simulink model "ADCS"  (R2018b)
settings: Solver=VariableStepAuto  StartTime=0.0  StopTime=10  RelTol=1e-3
undefined symbols (not defined in the file): f, Jw, Kb, km, Kt, La, N, Ra, tau
libraries: vrlib x1
settings Model: Creator=mario  LastModifiedBy=mario

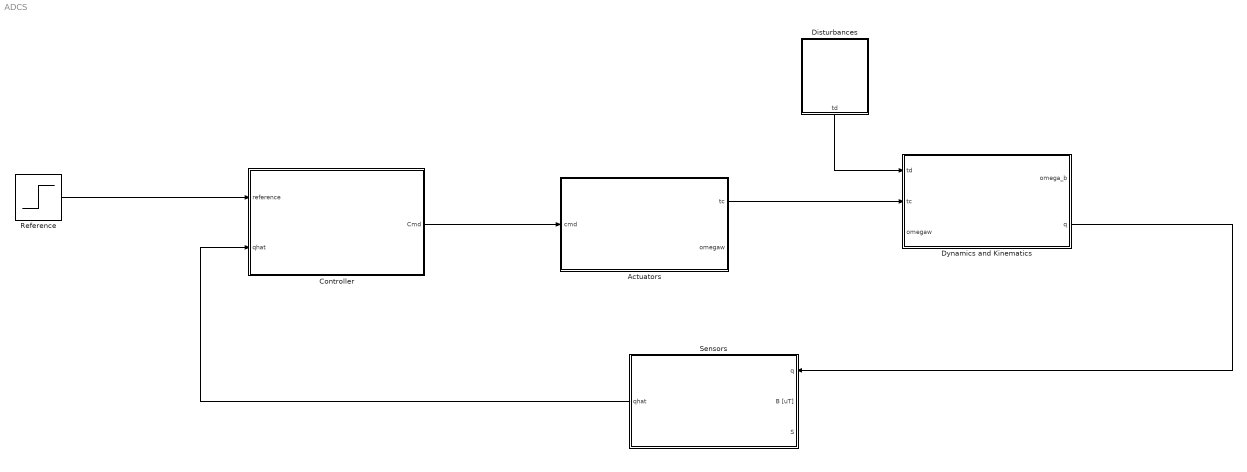
== system ADCS ==
  Actuators : Subsystem
  Controller : Subsystem
  Disturbances : Subsystem
  "Dynamics and Kinematics " : Subsystem
  Reference : Step  SampleTime=0
  Sensors : Subsystem
  wires:
  "Dynamics and Kinematics "/2(q) -> Sensors/1(q)
  Sensors/1(qhat) -> Controller/2(qhat)
  Controller/1(Cmd) -> Actuators/1(cmd)
  Disturbances/1(td) -> "Dynamics and Kinematics "/1(td)
  Actuators/1(tc) -> "Dynamics and Kinematics "/2(tc)
  Reference/1 -> Controller/1("reference ")

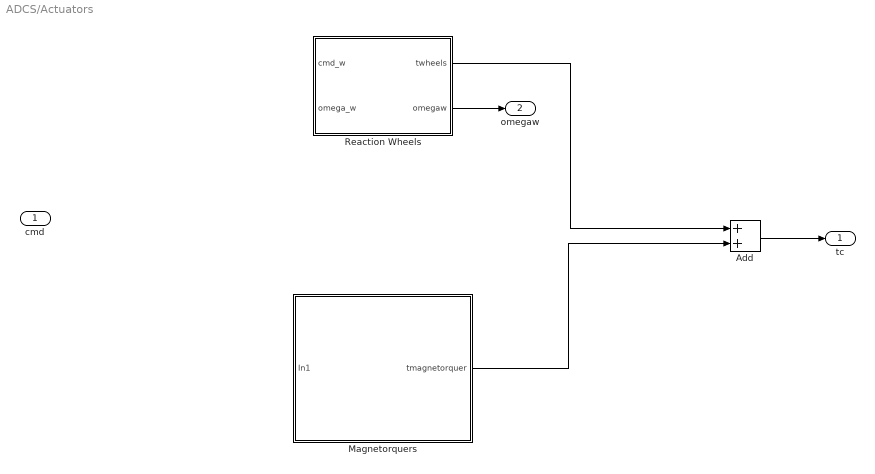
== system ADCS/Actuators ==
  cmd : Inport
  Add : Sum
  Magnetorquers : Subsystem
  Reaction Wheels : Subsystem
  tc : Outport
  omegaw : Outport  Port=2
  wires:
  Reaction Wheels/1(twheels) -> Add/1
  Magnetorquers/1(tmagnetorquer) -> Add/2
  Add/1 -> tc/1
  Reaction Wheels/2(omegaw) -> omegaw/1

== system ADCS/Controller ==
  "reference " : Inport
  qhat : Inport  Port=2
  Cmd : Outport

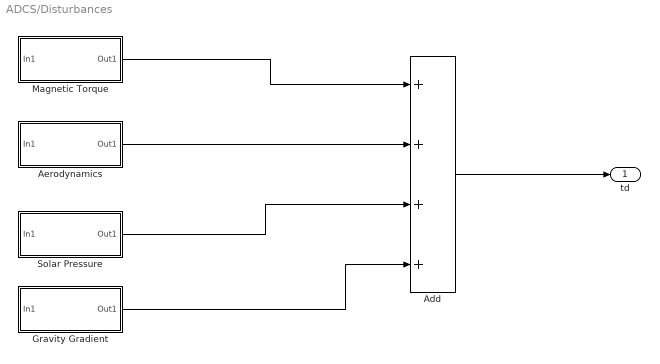
== system ADCS/Disturbances ==
  Add : Sum  Inputs=4
  Aerodynamics : Subsystem
  Gravity Gradient : Subsystem
  Magnetic Torque : Subsystem
  Solar Pressure : Subsystem
  td : Outport
  wires:
  Add/1 -> td/1
  Magnetic Torque/1(Out1) -> Add/1
  Aerodynamics/1(Out1) -> Add/2
  Solar Pressure/1(Out1) -> Add/3
  Gravity Gradient/1(Out1) -> Add/4

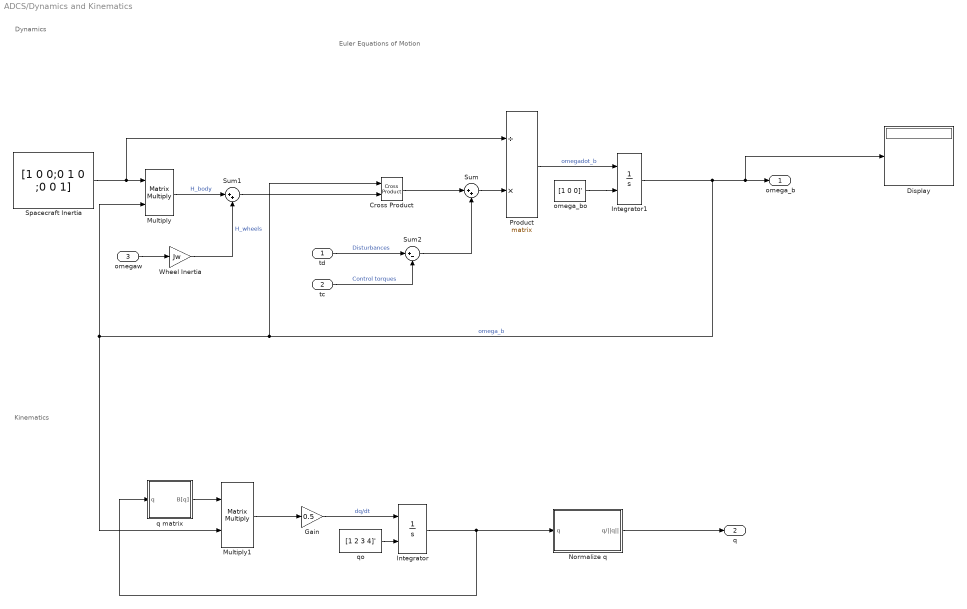
== system ADCS/Dynamics and Kinematics  ==
  note: Kinematics
  note: Dynamics
  note: Euler Equations of Motion
  td : Inport
  tc : Inport  Port=2
  omegaw : Inport  Port=3
  Cross Product : vrlib/Utilities/Cross Product
      settings: SourceProductBaseCode=VR
  Display : Display
  Gain : Gain  Gain=0.5
  Integrator : Integrator  InitialConditionSource=external
  Integrator1 : Integrator  InitialConditionSource=external
  Multiply : Product  Multiplication=Matrix(*)
  Multiply1 : Product  Multiplication=Matrix(*)
  Normalize q : Subsystem
  Product : Product  Inputs=/*  Multiplication=Matrix(*)
  Spacecraft Inertia : Constant  Value=[1 0 0;0 1 0 ;0 0 1]
  Sum : Sum  Inputs=|++
  Sum1 : Sum  Inputs=|++
  Sum2 : Sum  Inputs=|+-
  Wheel Inertia : Gain  Gain=Jw
  omega_bo : Constant  Value=[1 0 0]'
  q matrix : Subsystem
  qo : Constant  Value=[1 2 3 4]'
  omega_b : Outport
  q : Outport  Port=2
  wires:
  Integrator1/1 -> Display/1, omega_b/1, Multiply1/2, Multiply/2, Cross Product/1  "omega_b"
  Spacecraft Inertia/1 -> Product/1, Multiply/1
  omega_bo/1 -> Integrator1/2
  Product/1 -> Integrator1/1  "omegadot_b"
  Multiply/1 -> Sum1/1  "H_body"
  Sum/1 -> Product/2
  Cross Product/1 -> Sum/1
  Sum1/1 -> Cross Product/2
  Wheel Inertia/1 -> Sum1/2  "H_wheels"
  omegaw/1 -> Wheel Inertia/1
  td/1 -> Sum2/1  "Disturbances"
  tc/1 -> Sum2/2  "Control torques"
  Sum2/1 -> Sum/2
  Multiply1/1 -> Gain/1
  Gain/1 -> Integrator/1  "dq/dt"
  Integrator/1 -> Normalize q/1(q), q matrix/1(q)
  q matrix/1(B[q]) -> Multiply1/1
  qo/1 -> Integrator/2
  Normalize q/1(q/||q||) -> q/1

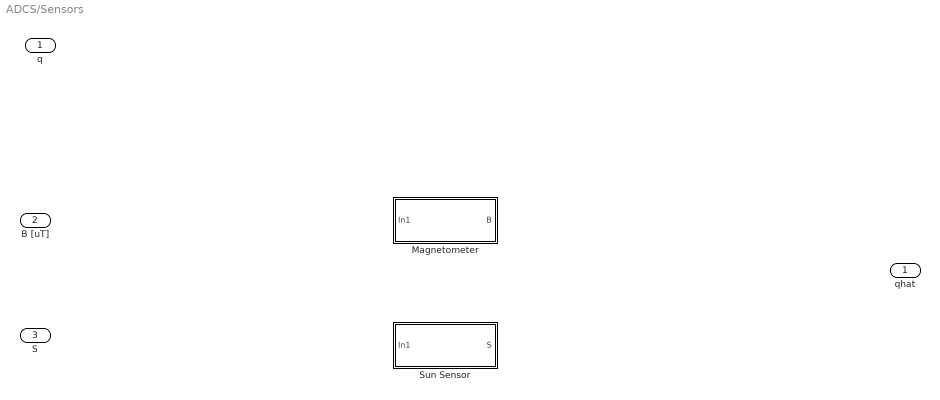
== system ADCS/Sensors ==
  q : Inport
  B [uT] : Inport  Port=2
  S : Inport  Port=3
  Magnetometer : Subsystem
  Sun Sensor : Subsystem
  qhat : Outport

== system ADCS/Actuators/Magnetorquers ==
  In1 : Inport
  tmagnetorquer : Outport
  wires:
  In1/1 -> tmagnetorquer/1

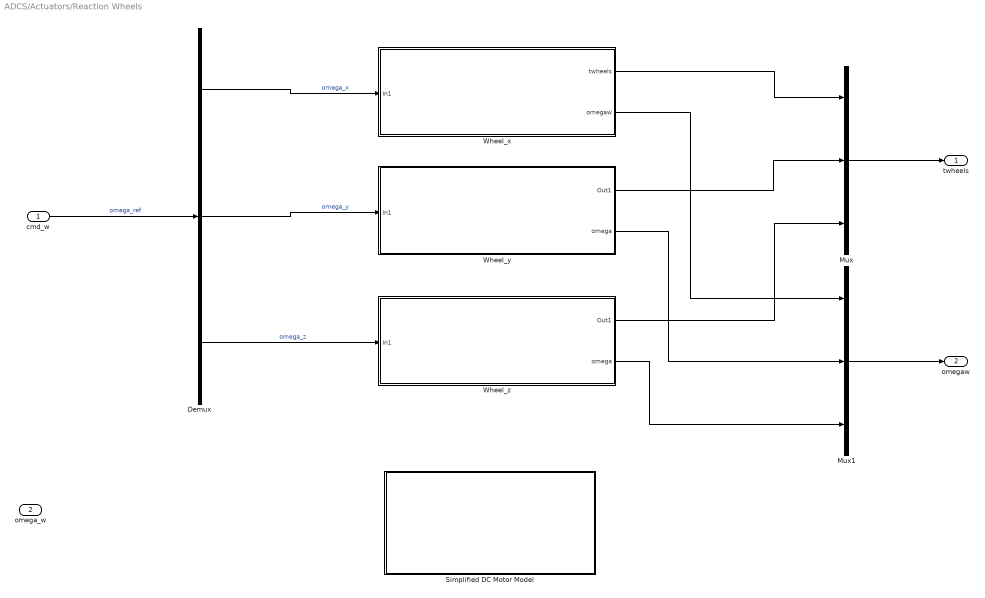
== system ADCS/Actuators/Reaction Wheels ==
  cmd_w : Inport
  omega_w : Inport  Port=2
  Demux : Demux  Outputs=3
  Mux : Mux  Inputs=3
  Mux1 : Mux  Inputs=3
  Simplified DC Motor Model : Subsystem
  Wheel_x : Subsystem
  Wheel_y : Subsystem
  Wheel_z : Subsystem
  twheels : Outport
  omegaw : Outport  Port=2
  wires:
  cmd_w/1 -> Demux/1  "omega_ref"
  Wheel_x/1(twheels) -> Mux/1
  Wheel_x/2(omegaw) -> Mux1/1
  Demux/3 -> Wheel_z/1(In1)  "omega_z"
  Demux/2 -> Wheel_y/1(In1)  "omega_y"
  Demux/1 -> Wheel_x/1(In1)  "omega_x"
  Mux/1 -> twheels/1
  Wheel_y/1(Out1) -> Mux/2
  Wheel_z/1(Out1) -> Mux/3
  Wheel_y/2(omega) -> Mux1/2
  Wheel_z/2(omega) -> Mux1/3
  Mux1/1 -> omegaw/1

== system ADCS/Disturbances/Aerodynamics ==
  In1 : Inport
  Out1 : Outport

== system ADCS/Disturbances/Gravity Gradient ==
  In1 : Inport
  Out1 : Outport
  wires:
  In1/1 -> Out1/1

== system ADCS/Disturbances/Magnetic Torque ==
  In1 : Inport
  Out1 : Outport
  wires:
  In1/1 -> Out1/1

== system ADCS/Disturbances/Solar Pressure ==
  In1 : Inport
  Out1 : Outport
  wires:
  In1/1 -> Out1/1

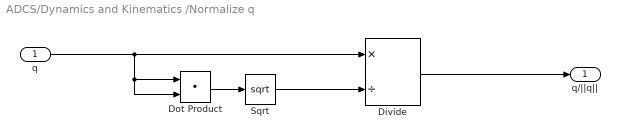
== system ADCS/Dynamics and Kinematics /Normalize q ==
  q : Inport
  Divide : Product  Inputs=*/
  Dot Product : DotProduct  InputSameDT=on  OutDataTypeStr=Inherit: Inherit via internal rule
  Sqrt : Sqrt  SaturateOnIntegerOverflow=on
  q/||q|| : Outport
  wires:
  q/1 -> Divide/1, Dot Product/2, Dot Product/1
  Sqrt/1 -> Divide/2
  Dot Product/1 -> Sqrt/1
  Divide/1 -> q/||q||/1

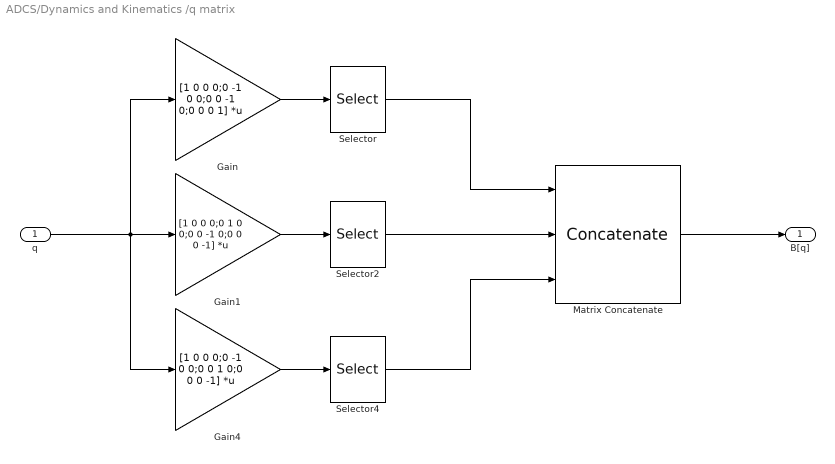
== system ADCS/Dynamics and Kinematics /q matrix ==
  q : Inport
  Gain : Gain  Gain=[1 0 0 0;0 -1 0 0;0 0 -1 0;0 0 0 1]  Multiplication=Matrix(K*u)
  Gain1 : Gain  Gain=[1 0 0 0;0 1 0 0;0 0 -1 0;0 0 0 -1]  Multiplication=Matrix(K*u)
  Gain4 : Gain  Gain=[1 0 0 0;0 -1 0 0;0 0 1 0;0 0 0 -1]  Multiplication=Matrix(K*u)
  Matrix Concatenate : Concatenate  NumInputs=3  Mode=Multidimensional array  ConcatenateDimension=2
  Selector : Selector  InputPortWidth=4  IndexOptions=Index vector (dialog)  Indices=[2 1 4 3]  OutputSizes=1
  Selector2 : Selector  InputPortWidth=4  IndexOptions=Index vector (dialog)  Indices=[3 4 1 2]  OutputSizes=1
  Selector4 : Selector  InputPortWidth=4  IndexOptions=Index vector (dialog)  Indices=[4 3 2 1]  OutputSizes=1
  B[q] : Outport
  wires:
  Gain4/1 -> Selector4/1
  Selector2/1 -> Matrix Concatenate/2
  Matrix Concatenate/1 -> B[q]/1
  Selector4/1 -> Matrix Concatenate/3
  q/1 -> Gain4/1, Gain/1, Gain1/1
  Selector/1 -> Matrix Concatenate/1
  Gain1/1 -> Selector2/1
  Gain/1 -> Selector/1

== system ADCS/Sensors/Magnetometer ==
  In1 : Inport
  B : Outport

== system ADCS/Sensors/Sun Sensor ==
  In1 : Inport
  S : Outport

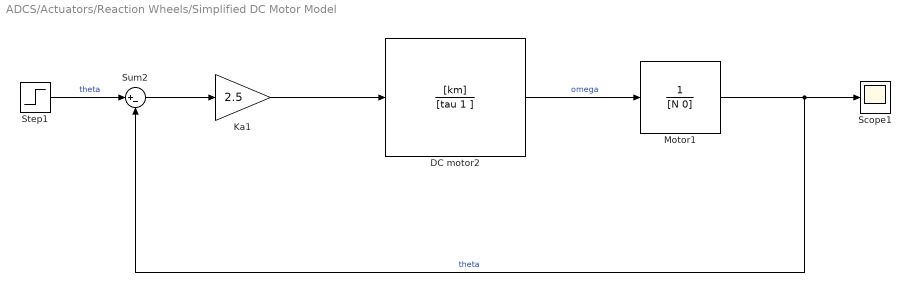
== system ADCS/Actuators/Reaction Wheels/Simplified DC Motor Model ==
  DC motor2 : TransferFcn  Numerator=[km]  Denominator=[tau 1 ]
  Ka1 : Gain  Gain=2.5
  Motor1 : TransferFcn  Denominator=[N 0]
  Scope1 : Scope
  Step1 : Step  Time=0  SampleTime=0
  Sum2 : Sum  Inputs=|+-
  wires:
  Step1/1 -> Sum2/1  "theta"
  Sum2/1 -> Ka1/1
  Ka1/1 -> DC motor2/1
  Motor1/1 -> Sum2/2, Scope1/1  "theta"
  DC motor2/1 -> Motor1/1  "omega"

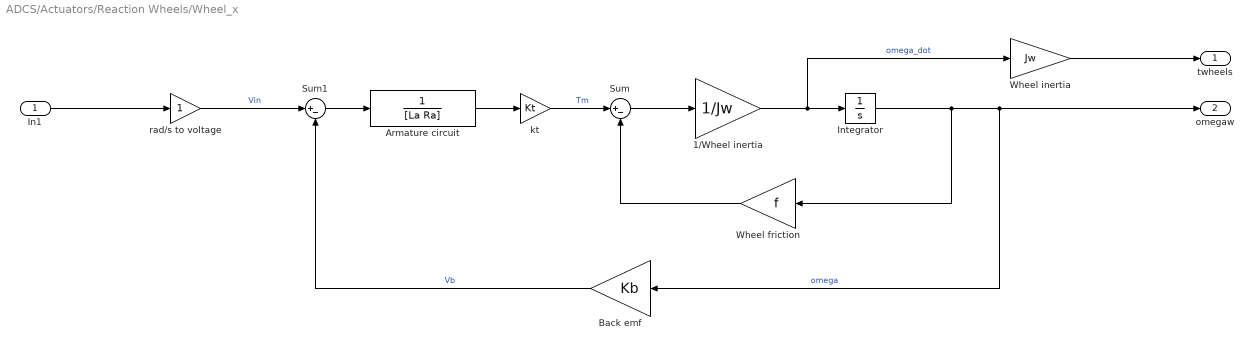
== system ADCS/Actuators/Reaction Wheels/Wheel_x ==
  In1 : Inport
  1/Wheel inertia : Gain  Gain=1/Jw
  Armature circuit : TransferFcn  Denominator=[La Ra]
  Back emf : Gain  Gain=Kb
  Integrator : Integrator
  Sum : Sum  Inputs=|+-
  Sum1 : Sum  Inputs=|+-
  Wheel friction : Gain  Gain=f
  Wheel inertia : Gain  Gain=Jw
  kt : Gain  Gain=Kt
  rad/s to voltage : Gain
  twheels : Outport
  omegaw : Outport  Port=2
  wires:
  rad/s to voltage/1 -> Sum1/1  "Vin"
  Back emf/1 -> Sum1/2  "Vb"
  Sum/1 -> 1/Wheel inertia/1
  kt/1 -> Sum/1  "Tm"
  1/Wheel inertia/1 -> Wheel inertia/1, Integrator/1  "omega_dot"
  Sum1/1 -> Armature circuit/1
  Wheel friction/1 -> Sum/2
  Integrator/1 -> Wheel friction/1, omegaw/1, Back emf/1  "omega"
  Armature circuit/1 -> kt/1
  Wheel inertia/1 -> twheels/1
  In1/1 -> rad/s to voltage/1

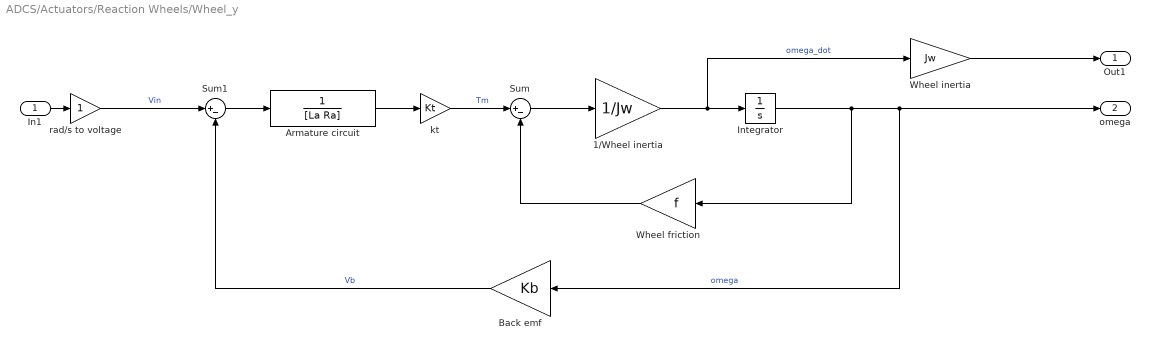
== system ADCS/Actuators/Reaction Wheels/Wheel_y ==
  In1 : Inport
  1/Wheel inertia : Gain  Gain=1/Jw
  Armature circuit : TransferFcn  Denominator=[La Ra]
  Back emf : Gain  Gain=Kb
  Integrator : Integrator
  Sum : Sum  Inputs=|+-
  Sum1 : Sum  Inputs=|+-
  Wheel friction : Gain  Gain=f
  Wheel inertia : Gain  Gain=Jw
  kt : Gain  Gain=Kt
  rad/s to voltage : Gain
  Out1 : Outport
  omega : Outport  Port=2
  wires:
  rad/s to voltage/1 -> Sum1/1  "Vin"
  Back emf/1 -> Sum1/2  "Vb"
  Sum/1 -> 1/Wheel inertia/1
  kt/1 -> Sum/1  "Tm"
  1/Wheel inertia/1 -> Wheel inertia/1, Integrator/1  "omega_dot"
  Sum1/1 -> Armature circuit/1
  Wheel friction/1 -> Sum/2
  Integrator/1 -> Wheel friction/1, omega/1, Back emf/1  "omega"
  Armature circuit/1 -> kt/1
  Wheel inertia/1 -> Out1/1
  In1/1 -> rad/s to voltage/1

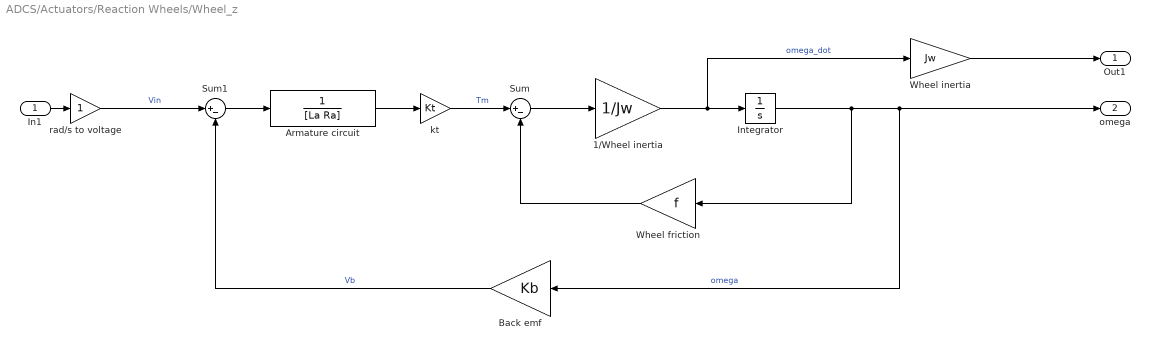
== system ADCS/Actuators/Reaction Wheels/Wheel_z ==
  In1 : Inport
  1/Wheel inertia : Gain  Gain=1/Jw
  Armature circuit : TransferFcn  Denominator=[La Ra]
  Back emf : Gain  Gain=Kb
  Integrator : Integrator
  Sum : Sum  Inputs=|+-
  Sum1 : Sum  Inputs=|+-
  Wheel friction : Gain  Gain=f
  Wheel inertia : Gain  Gain=Jw
  kt : Gain  Gain=Kt
  rad/s to voltage : Gain
  Out1 : Outport
  omega : Outport  Port=2
  wires:
  rad/s to voltage/1 -> Sum1/1  "Vin"
  Back emf/1 -> Sum1/2  "Vb"
  Sum/1 -> 1/Wheel inertia/1
  kt/1 -> Sum/1  "Tm"
  1/Wheel inertia/1 -> Wheel inertia/1, Integrator/1  "omega_dot"
  Sum1/1 -> Armature circuit/1
  Wheel friction/1 -> Sum/2
  Integrator/1 -> Wheel friction/1, omega/1, Back emf/1  "omega"
  Armature circuit/1 -> kt/1
  Wheel inertia/1 -> Out1/1
  In1/1 -> rad/s to voltage/1
